simulink model "step_test"  (Simulink 9.3)
settings: Solver=VariableStepAuto  StartTime=0.0  StopTime=590  RelTol=1e-3  EnableMultiTasking=on
StartFcn:
  | clear all
libraries: realtime_pacer_lib x1
settings Model: Creator=johnh  LastModifiedBy=hgarnier
settings DataIOCC: SaveFormat=Dataset  SignalLoggingSaveFormat=Dataset
settings DebuggingCC: UnderspecifiedInitializationDetection=Simplified  MergeDetectMultiDrivingBlocksExec=error  FcnCallInpInsideContextMsg=error  PregeneratedLibrarySubsystemCodeDiagnostic=none
settings HardwareCC: ProdBitPerPointer=64  ProdBitPerSizeT=64  ProdBitPerPtrDiffT=64  ProdLargestAtomicFloat=Float  ProdIntDivRoundTo=Zero  ProdEndianess=LittleEndian  ProdWordSize=64  ProdHWDeviceType=Intel->x86-64 (Windows64)
settings ModelReferenceCC: PropagateSignalLabelsOutOfModel=on
settings GRTTargetCC: GeneratePreprocessorConditionals=Disable all  CombineOutputUpdateFcns=on  GRTInterface=off

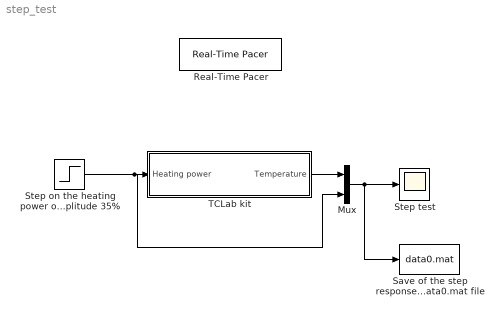
== system step_test ==
  Mux : Mux  Inputs=2
  Real-Time Pacer : realtime_pacer_lib/Real-Time Pacer  simTimePerRealTime=1
  Save of the step response data  in the data0.mat file : ToFile  Filename=data0.mat  MatrixName=data0
  Step on the heating power of amplitude 35% : Step  Time=25  After=35  SampleTime=0
  Step test : Scope
  TCLab kit : Subsystem
  wires:
  Step on the heating power of amplitude 35%/1 -> Mux/2, TCLab kit/1(Heating power)
  TCLab kit/1(Temperature) -> Mux/1
  Mux/1 -> Save of the step response data  in the data0.mat file/1, Step test/1

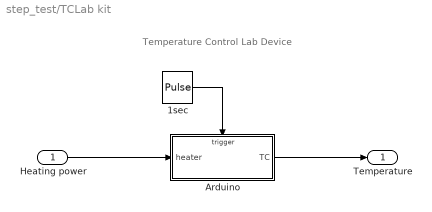
== system step_test/TCLab kit ==
  note: Temperature Control Lab Device
  Heating power : Inport
  1sec : DiscretePulseGenerator  PulseType=Time based  Period=1  PulseWidth=50
  Arduino : Subsystem  TreatAsAtomicUnit=on
  Temperature : Outport
  wires:
  1sec/1 -> Arduino/Trigger
  Arduino/1(TC) -> Temperature/1
  Heating power/1 -> Arduino/1(heater)

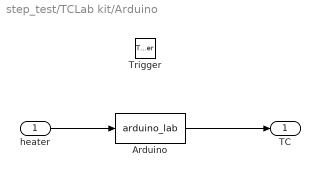
== system step_test/TCLab kit/Arduino ==
  heater : Inport
  Trigger : TriggerPort  VariantControl=Variant
  Arduino : MATLABFcn  MATLABFcn=arduino_lab
  TC : Outport  InitialOutput=23
  wires:
  heater/1 -> Arduino/1
  Arduino/1 -> TC/1
